simulink model "citt_generated_model_tevc"  (R2026b)
settings: Solver=ode23t  StopTime=1
undefined symbols (not defined in the file): R_e
libraries: fl_lib x11, nesl_utility x4, ee_lib x4
settings Model: Creator=Raalm  LastModifiedBy=Raalm
settings SimscapeCC: SimscapeLogType=all  SimscapeNominalValues="[{\"value\":\"1\",\"unit\":\"A\"},{\"value\":\"1\",\"unit\":\"bar\"},{\"value\":\"1\",\"unit\":\"cm^2\"},{\"value\":\"1\",\"unit\":\"cm^3/s\"},{\"value\":\"1\",\"unit\":\"kJ/kg\"},{\"value\":\"1\",\"unit\":\"kW\"},{\"value\":\"1\",\"unit\":\"l\"},{\"value\":\"1\",\"unit\":\"N\"},{\"value\":\"1\",\"unit\":\"N*m\"},{\"value\":\"1\",\"unit\":\"V\"},{\"value\":\"0.001\",\"unit\":\"Wb\"}]"  SimscapeUseEnergyAccounting=off

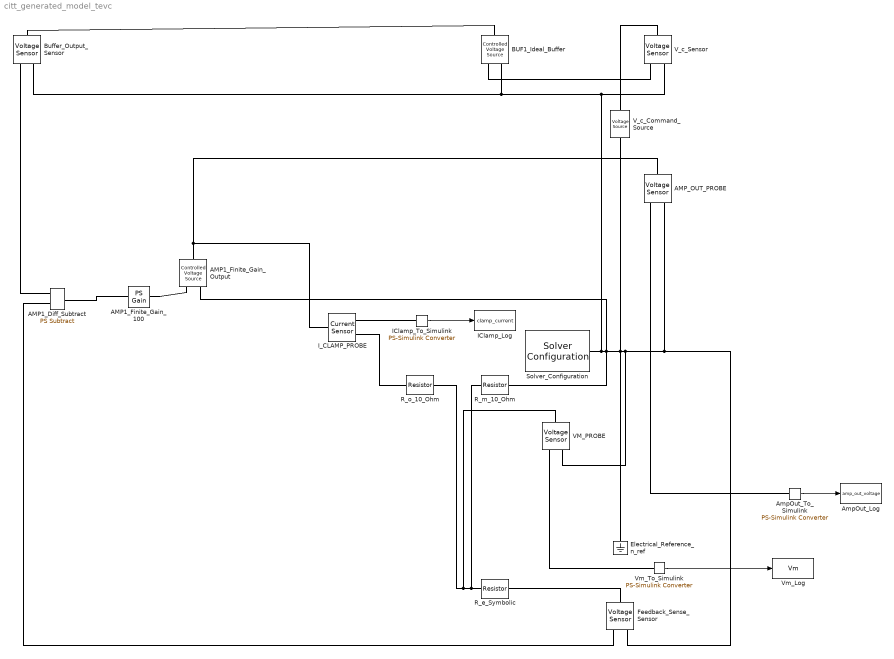
== system citt_generated_model_tevc ==
  AMP1_Diff_Subtract : fl_lib/Physical Signals/Functions/PS Subtract
  AMP1_Finite_Gain_100 : fl_lib/Physical Signals/Functions/PS Gain  gain=100
  AMP1_Finite_Gain_Output : fl_lib/Electrical/Electrical Sources/Controlled Voltage Source
  AMP_OUT_PROBE : fl_lib/Electrical/Electrical Sensors/Voltage Sensor
  AmpOut_Log : ToWorkspace  VariableName=amp_out_voltage  SaveFormat=Timeseries  SampleTime=-1
  AmpOut_To_Simulink : nesl_utility/PS-Simulink Converter  PhysicalDomain=network_engine_domain  SubClassName=ps_output  LeftPortType=input  RightPortType=output  PseudoPeriodic=off  Frequencies=[]  VectorFormat=inherit  Unit=inherit  AffineConversion=off
  BUF1_Ideal_Buffer : fl_lib/Electrical/Electrical Sources/Controlled Voltage Source
  Buffer_Output_Sensor : fl_lib/Electrical/Electrical Sensors/Voltage Sensor
  Electrical_Reference_n_ref : fl_lib/Electrical/Electrical Elements/Electrical Reference
  Feedback_Sense_Sensor : fl_lib/Electrical/Electrical Sensors/Voltage Sensor
  IClamp_Log : ToWorkspace  VariableName=clamp_current  SaveFormat=Timeseries  SampleTime=-1
  IClamp_To_Simulink : nesl_utility/PS-Simulink Converter  PhysicalDomain=network_engine_domain  SubClassName=ps_output  LeftPortType=input  RightPortType=output  PseudoPeriodic=off  Frequencies=[]  VectorFormat=inherit  Unit=inherit  AffineConversion=off
  I_CLAMP_PROBE : fl_lib/Electrical/Electrical Sensors/Current Sensor
  R_e_Symbolic : ee_lib/Passive/Resistor  R=R_e Ohm  enable_R_tol=ee.enum.toleranceApplication.none  R_tol=5  tol_distribution=ee.enum.toleranceDistribution.uniform  nSigma=4  enable_operating_limits=ee.enum.enable.no  operating_limit_action=ee.enum.passive.reportOpLim.warn  power_rating=1 W  max_working_voltage=100 V  noise_mode=ee.enum.sources.noise.Disabled  Tdevice=25 degC  sample_time=1e-3 s  repeatability=ee.enum.ic.repeatability.notRepeatable  user_seed=0  auto_seed=2288468478  power_derating_T1=70 degC  power_derating_T2=155 degC  operating_temperature_range_vec=[-50, 150] degC  alpha=3.93e-3 1/K  Tmeas=25 degC  thermal_mass=100 J/K  temperature_specify=off  temperature_priority=High  temperature=298.15 K  temperature_nominal_specify=off  temperature_nominal_value=1  temperature_nominal_unit=K
  R_m_10_Ohm : ee_lib/Passive/Resistor  R=10 Ohm  enable_R_tol=ee.enum.toleranceApplication.none  R_tol=5  tol_distribution=ee.enum.toleranceDistribution.uniform  nSigma=4  enable_operating_limits=ee.enum.enable.no  operating_limit_action=ee.enum.passive.reportOpLim.warn  power_rating=1 W  max_working_voltage=100 V  noise_mode=ee.enum.sources.noise.Disabled  Tdevice=25 degC  sample_time=1e-3 s  repeatability=ee.enum.ic.repeatability.notRepeatable  user_seed=0  auto_seed=3485711526  power_derating_T1=70 degC  power_derating_T2=155 degC  operating_temperature_range_vec=[-50, 150] degC  alpha=3.93e-3 1/K  Tmeas=25 degC  thermal_mass=100 J/K  temperature_specify=off  temperature_priority=High  temperature=298.15 K  temperature_nominal_specify=off  temperature_nominal_value=1  temperature_nominal_unit=K
  R_o_10_Ohm : ee_lib/Passive/Resistor  R=10 Ohm  enable_R_tol=ee.enum.toleranceApplication.none  R_tol=5  tol_distribution=ee.enum.toleranceDistribution.uniform  nSigma=4  enable_operating_limits=ee.enum.enable.no  operating_limit_action=ee.enum.passive.reportOpLim.warn  power_rating=1 W  max_working_voltage=100 V  noise_mode=ee.enum.sources.noise.Disabled  Tdevice=25 degC  sample_time=1e-3 s  repeatability=ee.enum.ic.repeatability.notRepeatable  user_seed=0  auto_seed=1626114917  power_derating_T1=70 degC  power_derating_T2=155 degC  operating_temperature_range_vec=[-50, 150] degC  alpha=3.93e-3 1/K  Tmeas=25 degC  thermal_mass=100 J/K  temperature_specify=off  temperature_priority=High  temperature=298.15 K  temperature_nominal_specify=off  temperature_nominal_value=1  temperature_nominal_unit=K
  Solver_Configuration : nesl_utility/Solver Configuration  PhysicalDomain=network_engine_domain  SubClassName=solver  LeftPortType=input  RightPortType=generic  Tones=[]  Harmonics=[]  SimulateNoise=off  Profile=off  UseLocalSampling=off  EnableSwitchedLinearOptims=on  FrequencyDomain=off  UseCCode=off  RelTol=0.001  AbsTol=0.001  MinStep=1e-09  ToWorkspace=off  RevertToSquareIcSolve=off  NumHomotopyIterations=100  PhasorMode=off  PhasorModeNumHarmonics=1  ConsistencySolver=NEWTON_XTOL_AFTER_FTOL  CanonicalOrdering=CANONICAL  OptimizeIntermediates=OPTIMIZED  MulticoreSolverChoice=BACKWARD_EULER  IndexReductionMethod=DerivativeReplacement  DoDC=off  ResidualTolerance=1e-09  ConsistencyTolSource=GLOBAL  ConsistencyAbsTol=0.001  ConsistencyRelTol=0.001  ConsistencyTolFactor=0.001  UseLocalSolver=off  LocalSolverChoice=NE_BACKWARD_EULER_ADVANCER  ResolveIndetEquations=on  FunctionEvalNumThread=1  LocalSolverSampleTime=0.001  DoFixedCost=off  MaxNonlinIter=3  MaxModeIter=2  ComputeImpulses=off  ImpulseIterations=2  LinearAlgebra=auto  LinearAlgebraNumThread=0  EquationFormulation=NE_TIME_EF  DelaysMemoryBudget=1024  AutomaticFiltering=on  FilteringTimeConstant=0.001  PartitionStorageMethod=AS_NEEDED  PartitionMemoryBudget=1024  PartitionMethod=BALANCED  MultibodyUseLocalSolver=off  MultibodyLocalSolverChoice=ODE1  MultibodyLocalSolverSampleTime=0.001
  VM_PROBE : fl_lib/Electrical/Electrical Sensors/Voltage Sensor
  V_c_Command_Source : ee_lib/Sources/Voltage Source  dc_voltage=V_c V  ac_voltage=0 V  ac_shift=0 rad  ac_frequency=60 Hz  noise_mode=ee.enum.sources.noise.Disabled  PSD=0 V^2/Hz  sample_time=1e-3 s  repeatability=ee.enum.sources.repeatability.NotRepeatable  user_seed=0  auto_seed=2767325297  i_specify=off  i_priority=None  i=0 A  i_nominal_specify=off  i_nominal_value=1  i_nominal_unit=A  v_specify=off  v_priority=None  v=0 V  v_nominal_specify=off  v_nominal_value=1  v_nominal_unit=V
  V_c_Sensor : fl_lib/Electrical/Electrical Sensors/Voltage Sensor
  Vm_Log : ToWorkspace  VariableName=Vm  SaveFormat=Timeseries  SampleTime=-1
  Vm_To_Simulink : nesl_utility/PS-Simulink Converter  PhysicalDomain=network_engine_domain  SubClassName=ps_output  LeftPortType=input  RightPortType=output  PseudoPeriodic=off  Frequencies=[]  VectorFormat=inherit  Unit=inherit  AffineConversion=off
  wires:
  AmpOut_To_Simulink/1 -> AmpOut_Log/1
  Vm_To_Simulink/1 -> Vm_Log/1
  IClamp_To_Simulink/1 -> IClamp_Log/1
  connections:
  AMP_OUT_PROBE/RConn1 -- AmpOut_To_Simulink/LConn1
  VM_PROBE/RConn1 -- Vm_To_Simulink/LConn1
  I_CLAMP_PROBE/RConn1 -- IClamp_To_Simulink/LConn1
  R_m_10_Ohm/LConn1 -- R_o_10_Ohm/RConn1 -- VM_PROBE/LConn1 -- R_e_Symbolic/LConn1
  I_CLAMP_PROBE/RConn2 -- R_o_10_Ohm/LConn1
  AMP_OUT_PROBE/LConn1 -- AMP1_Finite_Gain_Output/LConn1 -- I_CLAMP_PROBE/LConn1
  AMP1_Finite_Gain_100/RConn1 -- AMP1_Finite_Gain_Output/RConn1
  AMP1_Diff_Subtract/RConn1 -- AMP1_Finite_Gain_100/LConn1
  Feedback_Sense_Sensor/RConn1 -- AMP1_Diff_Subtract/LConn2
  R_e_Symbolic/RConn1 -- Feedback_Sense_Sensor/LConn1
  Buffer_Output_Sensor/RConn1 -- AMP1_Diff_Subtract/LConn1
  BUF1_Ideal_Buffer/LConn1 -- Buffer_Output_Sensor/LConn1
  V_c_Sensor/RConn1 -- BUF1_Ideal_Buffer/RConn1
  V_c_Command_Source/LConn1 -- V_c_Sensor/LConn1
  AMP_OUT_PROBE/RConn2 -- Buffer_Output_Sensor/RConn2 -- BUF1_Ideal_Buffer/RConn2 -- V_c_Sensor/RConn2 -- Solver_Configuration/RConn1 -- R_m_10_Ohm/RConn1 -- AMP1_Finite_Gain_Output/RConn2 -- V_c_Command_Source/RConn1 -- Electrical_Reference_n_ref/LConn1 -- VM_PROBE/RConn2 -- Feedback_Sense_Sensor/RConn2
